simulink model "Grid_1"  (R2016b)
settings: Solver=ode3  StartTime=0.0  StopTime=10.0  RelTol=1e-3
values from neighbouring files (symbols this model uses):
  Ts = 80e-6*2    (= 0.00016)    [initSimScript.m]
undefined symbols (not defined in the file or in its folder): DiscIntNeverNeededParam
libraries: cables_lib x21, simulink x18, modbus_lib x15, powerlib x10, dynamic_load_lib x8, transformer_lib x6, discretizing x4
(part 2 of 3)

== system Grid_1/GenSet_1MVA_09082015/Simulated Generator Controller 900 kW/PQ control ==
  P_ref (pu) : Inport
  P (pu) : Inport  Port=2
  Q_ref (pu) : Inport  Port=3
  Q (pu) : Inport  Port=4
  Discrete PID Controller : simulink/Continuous/PID Controller  Controller=PID  TimeDomain=Discrete-time  SampleTime=-1  IntegratorMethod=Forward Euler  FilterMethod=Forward Euler  Form=Parallel  UseFilter=on  ControllerParametersSource=internal  P=0.001  I=1  D=0  N=10  InitialConditionSource=internal  InitialConditionForIntegrator=0  InitialConditionForFilter=0  ExternalReset=none  LimitOutput=on  UpperSaturationLimit=1.15  LowerSaturationLimit=0.85  LinearizeAsGain=off  AntiWindupMode=back-calculation  Kb=1  TrackingMode=off  Kt=1  PParamMin=[]  PParamMax=[]  IParamMin=[]  IParamMax=[]  DParamMin=[]  DParamMax=[]  NParamMin=[]  NParamMax=[]  KbParamMin=[]  KbParamMax=[]  KtParamMin=[]  KtParamMax=[]  POutMin=[]  POutMax=[]  IOutMin=[]  IOutMax=[]  DOutMin=[]  DOutMax=[]  NOutMin=[]  NOutMax=[]  KbOutMin=[]  KbOutMax=[]  KtOutMin=[]  KtOutMax=[]  IntegratorOutMin=[]  IntegratorOutMax=[]  FilterOutMin=[]  FilterOutMax=[]  SumOutMin=[]  SumOutMax=[]  SumI1OutMin=[]  SumI1OutMax=[]  SumI2OutMin=[]  SumI2OutMax=[]  SumI3OutMin=[]  SumI3OutMax=[]  SumDOutMin=[]  SumDOutMax=[]  SaturationOutMin=[]  SaturationOutMax=[]  IntegratorContinuousStateAttributes=''  IntegratorStateMustResolveToSignalObject=off  IntegratorRTWStateStorageClass=Auto  FilterContinuousStateAttributes=''  FilterStateMustResolveToSignalObject=off  FilterRTWStateStorageClass=Auto  DifferentiatorICPrevScaledInput=0  DifferentiatorOutMin=[]  DifferentiatorOutMax=[]
  Discrete PID Controller1 : simulink/Continuous/PID Controller  Controller=PID  TimeDomain=Discrete-time  SampleTime=-1  IntegratorMethod=Forward Euler  FilterMethod=Forward Euler  Form=Parallel  UseFilter=on  ControllerParametersSource=internal  P=1.2  I=2.5  D=0  N=10  InitialConditionSource=internal  InitialConditionForIntegrator=0  InitialConditionForFilter=0  ExternalReset=none  LimitOutput=on  UpperSaturationLimit=1.15  LowerSaturationLimit=0.85  LinearizeAsGain=off  AntiWindupMode=back-calculation  Kb=1  TrackingMode=off  Kt=1  PParamMin=[]  PParamMax=[]  IParamMin=[]  IParamMax=[]  DParamMin=[]  DParamMax=[]  NParamMin=[]  NParamMax=[]  KbParamMin=[]  KbParamMax=[]  KtParamMin=[]  KtParamMax=[]  POutMin=[]  POutMax=[]  IOutMin=[]  IOutMax=[]  DOutMin=[]  DOutMax=[]  NOutMin=[]  NOutMax=[]  KbOutMin=[]  KbOutMax=[]  KtOutMin=[]  KtOutMax=[]  IntegratorOutMin=[]  IntegratorOutMax=[]  FilterOutMin=[]  FilterOutMax=[]  SumOutMin=[]  SumOutMax=[]  SumI1OutMin=[]  SumI1OutMax=[]  SumI2OutMin=[]  SumI2OutMax=[]  SumI3OutMin=[]  SumI3OutMax=[]  SumDOutMin=[]  SumDOutMax=[]  SaturationOutMin=[]  SaturationOutMax=[]  IntegratorContinuousStateAttributes=''  IntegratorStateMustResolveToSignalObject=off  IntegratorRTWStateStorageClass=Auto  FilterContinuousStateAttributes=''  FilterStateMustResolveToSignalObject=off  FilterRTWStateStorageClass=Auto  DifferentiatorICPrevScaledInput=0  DifferentiatorOutMin=[]  DifferentiatorOutMax=[]
  Sum : Sum  Inputs=|-+
  Sum1 : Sum  Inputs=|-+
  w_ref (pu) : Outport
  V_ref (pu) : Outport  Port=2
  wires:
  Q_ref (pu)/1 -> Sum1/2
  Discrete PID Controller1/1 -> V_ref (pu)/1
  Q (pu)/1 -> Sum1/1
  Sum1/1 -> Discrete PID Controller1/1
  P_ref (pu)/1 -> Sum/2
  Discrete PID Controller/1 -> w_ref (pu)/1
  P (pu)/1 -> Sum/1
  Sum/1 -> Discrete PID Controller/1

== system Grid_1/GenSet_1MVA_09082015/Simulated Generator Controller 900 kW/PV control ==
  P_ref (pu) : Inport
  P (pu) : Inport  Port=2
  Discrete PID Controller : simulink/Continuous/PID Controller  Controller=PID  TimeDomain=Discrete-time  SampleTime=-1  IntegratorMethod=Forward Euler  FilterMethod=Forward Euler  Form=Parallel  UseFilter=on  ControllerParametersSource=internal  P=0.001  I=1  D=0  N=10  InitialConditionSource=internal  InitialConditionForIntegrator=0  InitialConditionForFilter=0  ExternalReset=none  LimitOutput=on  UpperSaturationLimit=1.15  LowerSaturationLimit=0.85  LinearizeAsGain=off  AntiWindupMode=back-calculation  Kb=1  TrackingMode=off  Kt=1  PParamMin=[]  PParamMax=[]  IParamMin=[]  IParamMax=[]  DParamMin=[]  DParamMax=[]  NParamMin=[]  NParamMax=[]  KbParamMin=[]  KbParamMax=[]  KtParamMin=[]  KtParamMax=[]  POutMin=[]  POutMax=[]  IOutMin=[]  IOutMax=[]  DOutMin=[]  DOutMax=[]  NOutMin=[]  NOutMax=[]  KbOutMin=[]  KbOutMax=[]  KtOutMin=[]  KtOutMax=[]  IntegratorOutMin=[]  IntegratorOutMax=[]  FilterOutMin=[]  FilterOutMax=[]  SumOutMin=[]  SumOutMax=[]  SumI1OutMin=[]  SumI1OutMax=[]  SumI2OutMin=[]  SumI2OutMax=[]  SumI3OutMin=[]  SumI3OutMax=[]  SumDOutMin=[]  SumDOutMax=[]  SaturationOutMin=[]  SaturationOutMax=[]  IntegratorContinuousStateAttributes=''  IntegratorStateMustResolveToSignalObject=off  IntegratorRTWStateStorageClass=Auto  FilterContinuousStateAttributes=''  FilterStateMustResolveToSignalObject=off  FilterRTWStateStorageClass=Auto  DifferentiatorICPrevScaledInput=0  DifferentiatorOutMin=[]  DifferentiatorOutMax=[]
  Sum : Sum  Inputs=|-+
  w_ref (pu) : Outport
  wires:
  Sum/1 -> Discrete PID Controller/1
  P (pu)/1 -> Sum/1
  Discrete PID Controller/1 -> w_ref (pu)/1
  P_ref (pu)/1 -> Sum/2

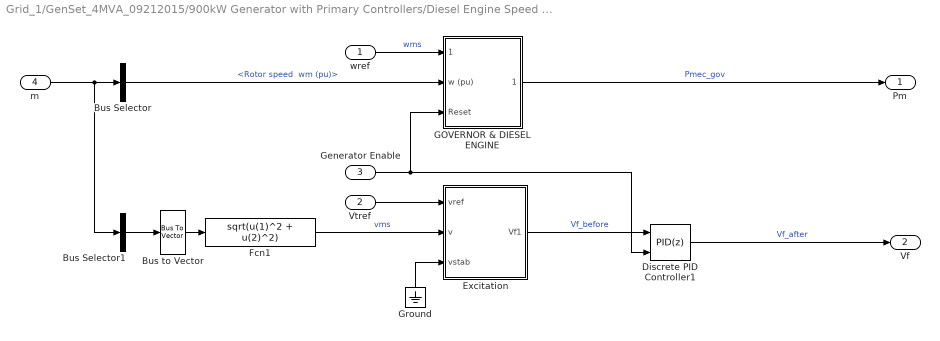
== system Grid_1/GenSet_4MVA_09212015/900kW Generator with Primary Controllers/Diesel Engine Speed & Voltage Control fast ==
  wref : Inport  SampleTime=Ts
  Vtref : Inport  Port=2  SampleTime=Ts
  Generator Enable : Inport  Port=3  SampleTime=Ts
  m : Inport  Port=4  SampleTime=Ts
  Bus Selector : BusSelector  OutputSignals="Mechanical.Rotor speed  wm (pu)"
  Bus Selector1 : BusSelector  OutputSignals="dq0 components.Stator voltage  vd (pu),dq0 components.Stator voltage  vq (pu)"  OutputAsBus=on
  Bus to Vector : BusToVector
  Discrete PID Controller1 : simulink/Continuous/PID Controller  Controller=PID  TimeDomain=Discrete-time  SampleTime=-1  IntegratorMethod=Forward Euler  FilterMethod=Forward Euler  Form=Parallel  UseFilter=on  ControllerParametersSource=internal  P=1  I=0  D=0  N=100  InitialConditionSource=internal  InitialConditionForIntegrator=0  InitialConditionForFilter=0  ExternalReset=either  LimitOutput=on  UpperSaturationLimit=5  LowerSaturationLimit=-5  LinearizeAsGain=off  AntiWindupMode=none  Kb=1  TrackingMode=off  Kt=1  PParamMin=[]  PParamMax=[]  IParamMin=[]  IParamMax=[]  DParamMin=[]  DParamMax=[]  NParamMin=[]  NParamMax=[]  KbParamMin=[]  KbParamMax=[]  KtParamMin=[]  KtParamMax=[]  POutMin=[]  POutMax=[]  IOutMin=[]  IOutMax=[]  DOutMin=[]  DOutMax=[]  NOutMin=[]  NOutMax=[]  KbOutMin=[]  KbOutMax=[]  KtOutMin=[]  KtOutMax=[]  IntegratorOutMin=[]  IntegratorOutMax=[]  FilterOutMin=[]  FilterOutMax=[]  SumOutMin=[]  SumOutMax=[]  SumI1OutMin=[]  SumI1OutMax=[]  SumI2OutMin=[]  SumI2OutMax=[]  SumI3OutMin=[]  SumI3OutMax=[]  SumDOutMin=[]  SumDOutMax=[]  SaturationOutMin=[]  SaturationOutMax=[]  IntegratorContinuousStateAttributes=''  IntegratorStateMustResolveToSignalObject=off  IntegratorRTWStateStorageClass=Auto  FilterContinuousStateAttributes=''  FilterStateMustResolveToSignalObject=off  FilterRTWStateStorageClass=Auto  DifferentiatorICPrevScaledInput=0  DifferentiatorOutMin=[]  DifferentiatorOutMax=[]
  Excitation : Subsystem  mask(Excitation System){tr=20e-4, reg=[ 200 2e-3 ], exc=[ 1 0.00000001 ], tgr=[ 1e-12 1e-12 ], damp=[0 1e-12 ], sat=[], lim=[ 0 5 0 ], v0=[ 0 0 ]}
      mask prompts: tr "Low-pass filter time constant Tr:"; reg "Regulator gain and time constant [ Ka  Ta ]:"; exc "Exciter  [ Ke  Te ]:"; tgr "Transient gain reduction [ Tb  Tc ]:"; damp "Damping filter gain and time constant  [ Kf  Tf  ]:"; sat "Field saturation parameters [ A B ]:"; lim "Regulator output limits and gain [ Efmin  Efmax  Kp ]:"; v0 "Initial values of terminal voltage  and field voltage [ Vt0 Vf0 ] :"
      mask help:
      | Implements an IEEE type 1 synchronous machine voltage regulator combined
      | to an exciter.
      |
      | The output of the block is the field voltage vfd, in pu,  to be applied to the Vf
      | Simulink input of a Synchronous Machine block.
      |
      | Connect the Vd and Vq measurements signals of the Synchronous Machine block
      | (signals 9 and 10)  to  the Vd and Vq inputs of the Excitation System block.
      mask Help: helpview(psbhelp);
  Fcn1 : Fcn  Expr=sqrt(u(1)^2 + u(2)^2)
  GOVERNOR & DIESEL ENGINE : Subsystem  mask(Diesel Engine & Governor){K=10, Ta=[0.025 0.0009 0.00574], Tlim=[0 1.1], Td=0.024, Pm0=0.0005}
      mask prompts: K "Regulator gain K:"; Ta "Actuator time constants [T4 T5 T6] (s) :"; Tlim "Torque limits [Tmin Tmax] (pu) :"; Td "Engine time delay Td (s) :"; Pm0 "Initial value of mechanical power  Pm0 (pu) :"
      mask help:
      | This block implements a diesel engine and governor system:
      | 1st and 2nd inputs: Desired and actual speed (pu)
      | Output: Diesel engine mechanical power.Motor inertia should be combined with generator.
      |
      | Actuator transfer function :
      |      Ha= (1+T4.s) / [ (s (1+T5.s)(1+T6.s) ]
      | Motor :
      |      Time delay Td
      |
      | (See reference in Tutorial Session 5)
  Ground : Ground
  Pm : Outport
  Vf : Outport  Port=2
  wires:
  GOVERNOR & DIESEL ENGINE/1(Pmec (pu)) -> Pm/1  "Pmec_gov"
  Generator Enable/1 -> GOVERNOR & DIESEL ENGINE/3(Reset), Discrete PID Controller1/2
  Bus to Vector/1 -> Fcn1/1
  Bus Selector1/1 -> Bus to Vector/1
  m/1 -> Bus Selector/1, Bus Selector1/1
  Bus Selector/1 -> GOVERNOR & DIESEL ENGINE/2(w (pu))  "<Rotor speed  wm (pu)>"
  Fcn1/1 -> Excitation/2(v)  "vms"
  Ground/1 -> Excitation/3(vstab)
  Excitation/1(Vf1) -> Discrete PID Controller1/1  "Vf_before"
  Discrete PID Controller1/1 -> Vf/1  "Vf_after"
  Vtref/1 -> Excitation/1(vref)
  wref/1 -> GOVERNOR & DIESEL ENGINE/1(wref (pu))  "wms"

== system Grid_1/GenSet_4MVA_09212015/Simulated Generator Controller 3.5 MW/PQ control ==
  P_ref (pu) : Inport
  P (pu) : Inport  Port=2
  Q_ref (pu) : Inport  Port=3
  Q (pu) : Inport  Port=4
  Discrete PID Controller : simulink/Continuous/PID Controller  Controller=PID  TimeDomain=Discrete-time  SampleTime=-1  IntegratorMethod=Forward Euler  FilterMethod=Forward Euler  Form=Parallel  UseFilter=on  ControllerParametersSource=internal  P=0.025  I=1  D=0  N=10  InitialConditionSource=internal  InitialConditionForIntegrator=0  InitialConditionForFilter=0  ExternalReset=none  LimitOutput=on  UpperSaturationLimit=1.15  LowerSaturationLimit=0.85  LinearizeAsGain=off  AntiWindupMode=back-calculation  Kb=1  TrackingMode=off  Kt=1  PParamMin=[]  PParamMax=[]  IParamMin=[]  IParamMax=[]  DParamMin=[]  DParamMax=[]  NParamMin=[]  NParamMax=[]  KbParamMin=[]  KbParamMax=[]  KtParamMin=[]  KtParamMax=[]  POutMin=[]  POutMax=[]  IOutMin=[]  IOutMax=[]  DOutMin=[]  DOutMax=[]  NOutMin=[]  NOutMax=[]  KbOutMin=[]  KbOutMax=[]  KtOutMin=[]  KtOutMax=[]  IntegratorOutMin=[]  IntegratorOutMax=[]  FilterOutMin=[]  FilterOutMax=[]  SumOutMin=[]  SumOutMax=[]  SumI1OutMin=[]  SumI1OutMax=[]  SumI2OutMin=[]  SumI2OutMax=[]  SumI3OutMin=[]  SumI3OutMax=[]  SumDOutMin=[]  SumDOutMax=[]  SaturationOutMin=[]  SaturationOutMax=[]  IntegratorContinuousStateAttributes=''  IntegratorStateMustResolveToSignalObject=off  IntegratorRTWStateStorageClass=Auto  FilterContinuousStateAttributes=''  FilterStateMustResolveToSignalObject=off  FilterRTWStateStorageClass=Auto  DifferentiatorICPrevScaledInput=0  DifferentiatorOutMin=[]  DifferentiatorOutMax=[]
  Discrete PID Controller1 : simulink/Continuous/PID Controller  Controller=PID  TimeDomain=Discrete-time  SampleTime=-1  IntegratorMethod=Forward Euler  FilterMethod=Forward Euler  Form=Parallel  UseFilter=on  ControllerParametersSource=internal  P=0.2  I=1.5  D=0  N=10  InitialConditionSource=internal  InitialConditionForIntegrator=0  InitialConditionForFilter=0  ExternalReset=none  LimitOutput=on  UpperSaturationLimit=1.15  LowerSaturationLimit=0.85  LinearizeAsGain=off  AntiWindupMode=back-calculation  Kb=1  TrackingMode=off  Kt=1  PParamMin=[]  PParamMax=[]  IParamMin=[]  IParamMax=[]  DParamMin=[]  DParamMax=[]  NParamMin=[]  NParamMax=[]  KbParamMin=[]  KbParamMax=[]  KtParamMin=[]  KtParamMax=[]  POutMin=[]  POutMax=[]  IOutMin=[]  IOutMax=[]  DOutMin=[]  DOutMax=[]  NOutMin=[]  NOutMax=[]  KbOutMin=[]  KbOutMax=[]  KtOutMin=[]  KtOutMax=[]  IntegratorOutMin=[]  IntegratorOutMax=[]  FilterOutMin=[]  FilterOutMax=[]  SumOutMin=[]  SumOutMax=[]  SumI1OutMin=[]  SumI1OutMax=[]  SumI2OutMin=[]  SumI2OutMax=[]  SumI3OutMin=[]  SumI3OutMax=[]  SumDOutMin=[]  SumDOutMax=[]  SaturationOutMin=[]  SaturationOutMax=[]  IntegratorContinuousStateAttributes=''  IntegratorStateMustResolveToSignalObject=off  IntegratorRTWStateStorageClass=Auto  FilterContinuousStateAttributes=''  FilterStateMustResolveToSignalObject=off  FilterRTWStateStorageClass=Auto  DifferentiatorICPrevScaledInput=0  DifferentiatorOutMin=[]  DifferentiatorOutMax=[]
  Sum : Sum  Inputs=|-+
  Sum1 : Sum  Inputs=|-+
  w_ref (pu) : Outport
  V_ref (pu) : Outport  Port=2
  wires:
  Q_ref (pu)/1 -> Sum1/2  "ref"
  Discrete PID Controller1/1 -> V_ref (pu)/1  "v"
  Q (pu)/1 -> Sum1/1  "pu"
  Sum1/1 -> Discrete PID Controller1/1  "dq"
  P_ref (pu)/1 -> Sum/2
  Discrete PID Controller/1 -> w_ref (pu)/1
  P (pu)/1 -> Sum/1
  Sum/1 -> Discrete PID Controller/1

== system Grid_1/GenSet_4MVA_09212015/Simulated Generator Controller 3.5 MW/PV control ==
  P_ref (pu) : Inport
  P (pu) : Inport  Port=2
  Discrete PID Controller : simulink/Continuous/PID Controller  Controller=PID  TimeDomain=Discrete-time  SampleTime=-1  IntegratorMethod=Forward Euler  FilterMethod=Forward Euler  Form=Parallel  UseFilter=on  ControllerParametersSource=internal  P=0.025  I=1  D=0  N=10  InitialConditionSource=internal  InitialConditionForIntegrator=0  InitialConditionForFilter=0  ExternalReset=none  LimitOutput=on  UpperSaturationLimit=1.15  LowerSaturationLimit=0.85  LinearizeAsGain=off  AntiWindupMode=back-calculation  Kb=1  TrackingMode=off  Kt=1  PParamMin=[]  PParamMax=[]  IParamMin=[]  IParamMax=[]  DParamMin=[]  DParamMax=[]  NParamMin=[]  NParamMax=[]  KbParamMin=[]  KbParamMax=[]  KtParamMin=[]  KtParamMax=[]  POutMin=[]  POutMax=[]  IOutMin=[]  IOutMax=[]  DOutMin=[]  DOutMax=[]  NOutMin=[]  NOutMax=[]  KbOutMin=[]  KbOutMax=[]  KtOutMin=[]  KtOutMax=[]  IntegratorOutMin=[]  IntegratorOutMax=[]  FilterOutMin=[]  FilterOutMax=[]  SumOutMin=[]  SumOutMax=[]  SumI1OutMin=[]  SumI1OutMax=[]  SumI2OutMin=[]  SumI2OutMax=[]  SumI3OutMin=[]  SumI3OutMax=[]  SumDOutMin=[]  SumDOutMax=[]  SaturationOutMin=[]  SaturationOutMax=[]  IntegratorContinuousStateAttributes=''  IntegratorStateMustResolveToSignalObject=off  IntegratorRTWStateStorageClass=Auto  FilterContinuousStateAttributes=''  FilterStateMustResolveToSignalObject=off  FilterRTWStateStorageClass=Auto  DifferentiatorICPrevScaledInput=0  DifferentiatorOutMin=[]  DifferentiatorOutMax=[]
  Sum : Sum  Inputs=|-+
  w_ref (pu) : Outport
  wires:
  Sum/1 -> Discrete PID Controller/1
  P (pu)/1 -> Sum/1
  Discrete PID Controller/1 -> w_ref (pu)/1
  P_ref (pu)/1 -> Sum/2

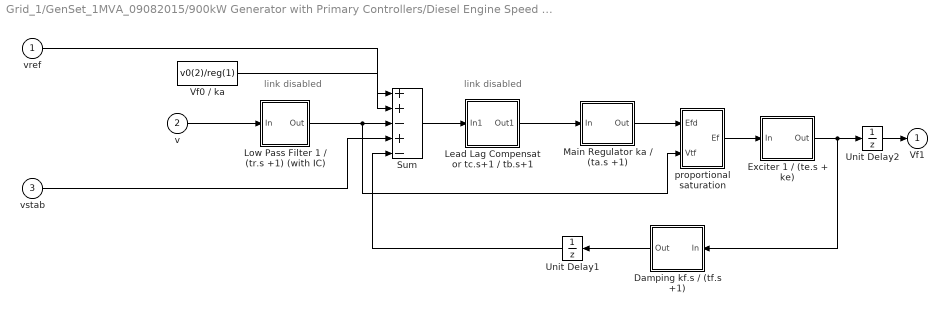
== system Grid_1/GenSet_1MVA_09082015/900kW Generator with Primary Controllers/Diesel Engine Speed & Voltage Control fast/Excitation ==
  note: link disabled
  note: link disabled
  vref : Inport
  v : Inport  Port=2
  vstab : Inport  Port=3
  Damping kf.s / (tf.s +1) : Subsystem
  Exciter 1 / (te.s + ke) : Subsystem
  Lead Lag Compensator tc.s+1 / tb.s+1 : Subsystem  AncestorBlock=|  mask(Discrete Lead-Lag Controller){T1=tgr(2), T2=tgr(1), V_Init=exc(1)*v0(2)/reg(1), Ts=Ts}
      | powerlib_extras/Discrete 
      | Control Blocks/Discrete
      | Lead-Lag
      mask prompts: T1 "Time constant T1 (s):"; T2 "Time constant T2 (s):"; V_Init "Initial input and output:"; Ts "Sample time (s):"
      mask help:
      | This block implements a discrete lead-lag controller:
      |
      |          1+T1s
      | H(s)= ------
      |          1+T2s
      |
      | States are initialized according to initial input anf output value so that simulation starts in steady state.
      mask init:
      | numc=[T1 1];
      | denc=[T2 1];
      | [Ac,Bc,Cc,Dc]=tf2ss(numc,denc);
      | 
      | %  Conversion to discrete transfer function
      | nstates = size(Ac,1);
      | invexp = inv(eye(nstates) - (Ts/2)*Ac);
      | Ad = invexp*(eye(nstates) + (Ts/2)*Ac);
      | Bd = invexp*Bc;
      | Cd = Cc*invexp*Ts;
      | Dd = Cc*invexp*Bc*(Ts/2) + Dc;
      | %
      | % Compute Initial states
      | I=eye(size(Ac));
      | x0c=inv(-Ac)*Bc*V_Init;
      | x0d=(I-Ac*Ts/2)*x0c/Ts - Bc/2*V_Init;
      | 
      | if T1==0 & T2==0, Dd=1; end
      mask Display: disp('1+T1s\n---\n1+T2s')
  Low Pass Filter 1 / (tr.s +1) (with IC) : Subsystem  AncestorBlock=|  mask(Discrete 1st-Order Filter){FilterType=Lowpass, Tc=tr, Ts=Ts, Initialize=on, Vac_Init=[0 0 60], Vdc_Init=v0(1), PlotResponse=off, param1=[1 500 0.1]}
      | powerlib_extras/Discrete 
      | Control Blocks/Discrete
      | 1st-Order
      | Discrete Filter
      mask prompts: FilterType "Filter Type:"; Tc "Time constant (s):"; Ts "Sample time:"; Initialize "Initialize filter states"; Vac_Init "AC initial input: [ Mag  Phase(degrees)  Freq(Hz) ]"; Vdc_Init "DC Initial input:"; PlotResponse "Plot filter response"; param1 "Frequency range(Hz) : [Start  End  Inc.]"
      mask init:
      | switch FilterType
      | case 1, % Lowpass
      |     X=[0 1 2 3 4];
      |     Y=[-2 -2 -3 -4 -4];
      |     numc=1;
      |     denc=[Tc 1];
      | case 2,   % Highpass
      |     X=[0 1 2 3 4];
      |     Y=[-4 -4 -3 -2 -2];
      |     numc=[1 0];
      |     denc=[1 1/Tc];
      | end
      | %
      | [Ac,Bc,Cc,Dc]=tf2ss(numc,denc);
      | %
      | %  Conversion to discrete transfer function
      | nstates = size(Ac,1);
      | invexp = inv(eye(nstates) - (Ts/2)*Ac);
      | Ad = invexp*(eye(nstates) + (Ts/2)*Ac);
      | Bd = invexp*Bc;
      | Cd = Cc*invexp*Ts;
      | Dd = Cc*invexp*Bc*(Ts/2) + Dc;
      | %
      | if Initialize==1  % Compute initial conditions on states
      |     u1=Vac_Init(1)*exp(j*Vac_Init(2)*pi/180);
      |     u2=Vdc_Init*exp(j*90*pi/180);
      |     u=u1+u2;
      |     u0=imag(u); % input at  t=0;
      |     I=eye(size(Ac));
      |     sI1=I*j*(2*pi*Vac_Init(3));
      |     sI2=I*j*0;
      |     x=inv(sI1-Ac)*Bc*u1 + inv(sI2-Ac)*Bc*u2;
      |     x0c=imag(x);
      |     x0d=(I-Ac*Ts/2)*x0c/Ts - Bc/2*u0;
      | else
      |     x0d=0;
      | end
      | 
      | %
      | if PlotResponse==1 % Plot frequency and step response
      |     figure(1)
      |     sys=ss(Ad,Bd,Cd,Dd,Ts);
      |     f=param1(1):param1(3):param1(2);
      |     w=2*pi*f;
      |     [mag phase]=bode(sys,w);
      |     subplot(2,1,1)
      |     plot(f,squeeze(mag))
      |     title('Magnitude')
      |     grid
      |     subplot(2,1,2)
      |     plot(f,squeeze(phase))
      |     title('Phase (degrees)')
      |     xlabel('Hz')
      |     grid
      |     figure(2)
      |     step(sys)
      | end
      mask TypeOptions FilterType: Lowpass | Highpass
      mask Callback Initialize: p4=get_param(gcb,'Initialize');if strcmp(p4,'on');visible={'on','on','on','on','on','on','on',get_param(gcb,'PlotResponse')};else;visible={'on','on','on','on','off','off','on',get_param(gcb,'PlotResponse')};end;set_param(gcb,'MaskVisibilities',visible)
      mask Callback PlotResponse: p7=get_param(gcb,'PlotResponse');if strcmp(p7,'on');visible={'on','on','on','on',get_param(gcb,'Initialize'),get_param(gcb,'Initialize'),'on','on'};else;visible={'on','on','on','on',get_param(gcb,'Initialize'),get_param(gcb,'Initialize'),'on','off'};end;set_param(gcb,'MaskVisibilities',visible)
      mask Display: plot(X,Y);
  Main Regulator ka / (ta.s +1) : Subsystem
  Sum : Sum  Inputs=++-+-  SaturateOnIntegerOverflow=on  InputSameDT=on  OutDataTypeStr=Inherit: Same as first input
  Unit Delay1 : UnitDelay  SampleTime=Ts
  Unit Delay2 : UnitDelay  InitialCondition=v0(2)  SampleTime=Ts
  Vf0 / ka : Constant  Value=v0(2)/reg(1)
  proportional saturation : Subsystem
  Vf1 : Outport
  wires:
  Exciter 1 / (te.s + ke)/1(Out) -> Damping kf.s / (tf.s +1)/1(In), Unit Delay2/1
  Damping kf.s / (tf.s +1)/1(Out) -> Unit Delay1/1
  Main Regulator ka / (ta.s +1)/1(Out) -> proportional saturation/1(Efd)
  Vf0 / ka/1 -> Sum/2
  Low Pass Filter 1 / (tr.s +1) (with IC)/1(Out) -> Sum/3, proportional saturation/2(Vtf)
  vstab/1 -> Sum/4
  vref/1 -> Sum/1
  v/1 -> Low Pass Filter 1 / (tr.s +1) (with IC)/1(In)
  Sum/1 -> Lead Lag Compensator tc.s+1 / tb.s+1/1(In1)
  Lead Lag Compensator tc.s+1 / tb.s+1/1(Out1) -> Main Regulator ka / (ta.s +1)/1(In)
  proportional saturation/1(Ef) -> Exciter 1 / (te.s + ke)/1(In)
  Unit Delay1/1 -> Sum/5
  Unit Delay2/1 -> Vf1/1

== system Grid_1/GenSet_1MVA_09082015/900kW Generator with Primary Controllers/Diesel Engine Speed & Voltage Control fast/GOVERNOR & DIESEL ENGINE ==
  note: ACTUATOR
  wref (pu) : Inport
  w (pu) : Inport  Port=2
  Reset : Inport  Port=3
  Discrete PID Controller : simulink/Continuous/PID Controller  Controller=PD  TimeDomain=Discrete-time  SampleTime=-1  IntegratorMethod=Forward Euler  FilterMethod=Forward Euler  Form=Parallel  UseFilter=on  ControllerParametersSource=internal  P=1  I=0  D=0.5  N=10000  InitialConditionSource=internal  InitialConditionForIntegrator=0  InitialConditionForFilter=0  ExternalReset=rising  ZeroCross=off  LimitOutput=off  UpperSaturationLimit=.5  LowerSaturationLimit=-.5  LinearizeAsGain=off  AntiWindupMode=none  Kb=1  TrackingMode=off  Kt=1  PParamMin=[]  PParamMax=[]  IParamMin=[]  IParamMax=[]  DParamMin=[]  DParamMax=[]  NParamMin=[]  NParamMax=[]  KbParamMin=[]  KbParamMax=[]  KtParamMin=[]  KtParamMax=[]  POutMin=[]  POutMax=[]  IOutMin=[]  IOutMax=[]  DOutMin=[]  DOutMax=[]  NOutMin=[]  NOutMax=[]  KbOutMin=[]  KbOutMax=[]  KtOutMin=[]  KtOutMax=[]  IntegratorOutMin=[]  IntegratorOutMax=[]  FilterOutMin=[]  FilterOutMax=[]  SumOutMin=[]  SumOutMax=[]  SumI1OutMin=[]  SumI1OutMax=[]  SumI2OutMin=[]  SumI2OutMax=[]  SumI3OutMin=[]  SumI3OutMax=[]  SumDOutMin=[]  SumDOutMax=[]  SaturationOutMin=[]  SaturationOutMax=[]  IntegratorContinuousStateAttributes=''  IntegratorStateMustResolveToSignalObject=off  IntegratorRTWStateStorageClass=Auto  FilterContinuousStateAttributes=''  FilterStateMustResolveToSignalObject=off  FilterRTWStateStorageClass=Auto  DifferentiatorICPrevScaledInput=0  DifferentiatorOutMin=[]  DifferentiatorOutMax=[]
  Discrete-Time Integrator : DiscreteIntegrator  IntegratorMethod=Integration: Backward Euler  ExternalReset=either  InitialCondition=Pm0  SampleTime=-1  LimitOutput=on  UpperSaturationLimit=Tlim(2)  LowerSaturationLimit=Tlim(1)  ICPrevOutput=DiscIntNeverNeededParam  ICPrevScaledInput=DiscIntNeverNeededParam
  ENGINE Td1 : TransportDelay  Commented=on  DelayTime=Td  InitialOutput=Pm0  BufferSize=7168
  Engine Delay : Delay  DelayLength=ceil(Td/Ts)  InitialCondition=Pm0
  Gain K : Gain  Gain=K  SaturateOnIntegerOverflow=on  OutDataTypeStr=Inherit: Same as input  ParamDataTypeStr=Inherit: Same as input
  Product : Product  SaturateOnIntegerOverflow=on  InputSameDT=on  OutDataTypeStr=Inherit: Same as first input
  Sum : Sum  Inputs=+-  SaturateOnIntegerOverflow=on  InputSameDT=on  OutDataTypeStr=Inherit: Same as first input
  TF3 : discretizing/Discretized Transfer Fcn  Numerator=1  Denominator=([Ta(3) 1])  AbsTol=auto  SampleTime=Ts  method=zoh  Wc=1
  TF4 : discretizing/Discretized Transfer Fcn  Numerator=([Ta(1) 1])  Denominator=([Ta(2) 1])  AbsTol=auto  SampleTime=Ts  method=zoh  Wc=1
  Pmec (pu) : Outport
  wires:
  Discrete PID Controller/1 -> Gain K/1
  Sum/1 -> Discrete PID Controller/1
  Gain K/1 -> TF4/1
  w (pu)/1 -> Product/2, Sum/2
  Engine Delay/1 -> Product/1
  wref (pu)/1 -> Sum/1
  Product/1 -> Pmec (pu)/1
  Discrete-Time Integrator/1 -> Engine Delay/1  "Torque"
  TF3/1 -> Discrete-Time Integrator/1
  TF4/1 -> TF3/1
  Reset/1 -> Discrete-Time Integrator/2, Discrete PID Controller/2

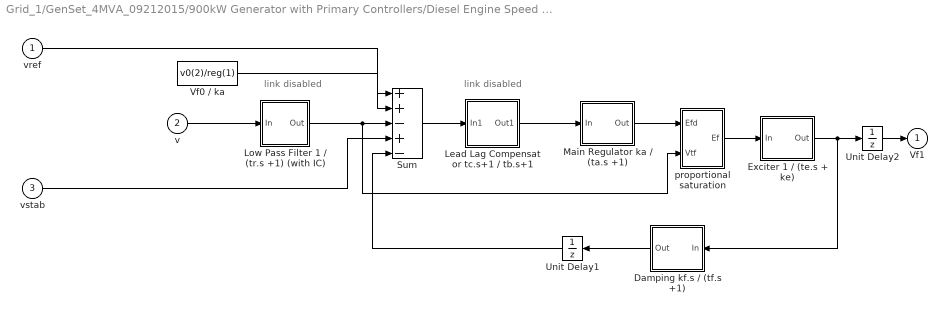
== system Grid_1/GenSet_4MVA_09212015/900kW Generator with Primary Controllers/Diesel Engine Speed & Voltage Control fast/Excitation ==
  note: link disabled
  note: link disabled
  vref : Inport
  v : Inport  Port=2
  vstab : Inport  Port=3
  Damping kf.s / (tf.s +1) : Subsystem
  Exciter 1 / (te.s + ke) : Subsystem
  Lead Lag Compensator tc.s+1 / tb.s+1 : Subsystem  AncestorBlock=|  mask(Discrete Lead-Lag Controller){T1=tgr(2), T2=tgr(1), V_Init=exc(1)*v0(2)/reg(1), Ts=Ts}
      | powerlib_extras/Discrete 
      | Control Blocks/Discrete
      | Lead-Lag
      mask prompts: T1 "Time constant T1 (s):"; T2 "Time constant T2 (s):"; V_Init "Initial input and output:"; Ts "Sample time (s):"
      mask help:
      | This block implements a discrete lead-lag controller:
      |
      |          1+T1s
      | H(s)= ------
      |          1+T2s
      |
      | States are initialized according to initial input anf output value so that simulation starts in steady state.
      mask init: same as Grid_1/GenSet_1MVA_09082015/900kW Generator with Primary Controllers/Diesel Engine Speed & Voltage Control fast/Excitation/Lead Lag Compensator tc.s+1 / tb.s+1
      mask Display: disp('1+T1s\n---\n1+T2s')
  Low Pass Filter 1 / (tr.s +1) (with IC) : Subsystem  AncestorBlock=|  mask(Discrete 1st-Order Filter){FilterType=Lowpass, Tc=tr, Ts=Ts, Initialize=on, Vac_Init=[0 0 60], Vdc_Init=v0(1), PlotResponse=off, param1=[1 500 0.1]}
      | powerlib_extras/Discrete 
      | Control Blocks/Discrete
      | 1st-Order
      | Discrete Filter
      mask prompts: FilterType "Filter Type:"; Tc "Time constant (s):"; Ts "Sample time:"; Initialize "Initialize filter states"; Vac_Init "AC initial input: [ Mag  Phase(degrees)  Freq(Hz) ]"; Vdc_Init "DC Initial input:"; PlotResponse "Plot filter response"; param1 "Frequency range(Hz) : [Start  End  Inc.]"
      mask init: same as Grid_1/GenSet_1MVA_09082015/900kW Generator with Primary Controllers/Diesel Engine Speed & Voltage Control fast/Excitation/Low Pass Filter 1 / (tr.s +1) (with IC)
      mask TypeOptions FilterType: Lowpass | Highpass
      mask Callback Initialize: p4=get_param(gcb,'Initialize');if strcmp(p4,'on');visible={'on','on','on','on','on','on','on',get_param(gcb,'PlotResponse')};else;visible={'on','on','on','on','off','off','on',get_param(gcb,'PlotResponse')};end;set_param(gcb,'MaskVisibilities',visible)
      mask Callback PlotResponse: p7=get_param(gcb,'PlotResponse');if strcmp(p7,'on');visible={'on','on','on','on',get_param(gcb,'Initialize'),get_param(gcb,'Initialize'),'on','on'};else;visible={'on','on','on','on',get_param(gcb,'Initialize'),get_param(gcb,'Initialize'),'on','off'};end;set_param(gcb,'MaskVisibilities',visible)
      mask Display: plot(X,Y);
  Main Regulator ka / (ta.s +1) : Subsystem
  Sum : Sum  Inputs=++-+-  SaturateOnIntegerOverflow=on  InputSameDT=on  OutDataTypeStr=Inherit: Same as first input
  Unit Delay1 : UnitDelay  SampleTime=Ts
  Unit Delay2 : UnitDelay  InitialCondition=v0(2)  SampleTime=Ts
  Vf0 / ka : Constant  Value=v0(2)/reg(1)
  proportional saturation : Subsystem
  Vf1 : Outport
  wires:
  Unit Delay2/1 -> Vf1/1
  Unit Delay1/1 -> Sum/5
  proportional saturation/1(Ef) -> Exciter 1 / (te.s + ke)/1(In)
  Lead Lag Compensator tc.s+1 / tb.s+1/1(Out1) -> Main Regulator ka / (ta.s +1)/1(In)
  Sum/1 -> Lead Lag Compensator tc.s+1 / tb.s+1/1(In1)
  v/1 -> Low Pass Filter 1 / (tr.s +1) (with IC)/1(In)
  vref/1 -> Sum/1
  vstab/1 -> Sum/4
  Low Pass Filter 1 / (tr.s +1) (with IC)/1(Out) -> proportional saturation/2(Vtf), Sum/3
  Vf0 / ka/1 -> Sum/2
  Main Regulator ka / (ta.s +1)/1(Out) -> proportional saturation/1(Efd)
  Damping kf.s / (tf.s +1)/1(Out) -> Unit Delay1/1
  Exciter 1 / (te.s + ke)/1(Out) -> Unit Delay2/1, Damping kf.s / (tf.s +1)/1(In)

== system Grid_1/GenSet_4MVA_09212015/900kW Generator with Primary Controllers/Diesel Engine Speed & Voltage Control fast/GOVERNOR & DIESEL ENGINE ==
  note: ACTUATOR
  wref (pu) : Inport
  w (pu) : Inport  Port=2
  Reset : Inport  Port=3
  Discrete PID Controller : simulink/Continuous/PID Controller  Controller=PD  TimeDomain=Discrete-time  SampleTime=-1  IntegratorMethod=Forward Euler  FilterMethod=Forward Euler  Form=Parallel  UseFilter=on  ControllerParametersSource=internal  P=1  I=0  D=0.5  N=10000  InitialConditionSource=internal  InitialConditionForIntegrator=0  InitialConditionForFilter=0  ExternalReset=rising  ZeroCross=off  LimitOutput=off  UpperSaturationLimit=.5  LowerSaturationLimit=-.5  LinearizeAsGain=off  AntiWindupMode=none  Kb=1  TrackingMode=off  Kt=1  PParamMin=[]  PParamMax=[]  IParamMin=[]  IParamMax=[]  DParamMin=[]  DParamMax=[]  NParamMin=[]  NParamMax=[]  KbParamMin=[]  KbParamMax=[]  KtParamMin=[]  KtParamMax=[]  POutMin=[]  POutMax=[]  IOutMin=[]  IOutMax=[]  DOutMin=[]  DOutMax=[]  NOutMin=[]  NOutMax=[]  KbOutMin=[]  KbOutMax=[]  KtOutMin=[]  KtOutMax=[]  IntegratorOutMin=[]  IntegratorOutMax=[]  FilterOutMin=[]  FilterOutMax=[]  SumOutMin=[]  SumOutMax=[]  SumI1OutMin=[]  SumI1OutMax=[]  SumI2OutMin=[]  SumI2OutMax=[]  SumI3OutMin=[]  SumI3OutMax=[]  SumDOutMin=[]  SumDOutMax=[]  SaturationOutMin=[]  SaturationOutMax=[]  IntegratorContinuousStateAttributes=''  IntegratorStateMustResolveToSignalObject=off  IntegratorRTWStateStorageClass=Auto  FilterContinuousStateAttributes=''  FilterStateMustResolveToSignalObject=off  FilterRTWStateStorageClass=Auto  DifferentiatorICPrevScaledInput=0  DifferentiatorOutMin=[]  DifferentiatorOutMax=[]
  Discrete-Time Integrator : DiscreteIntegrator  IntegratorMethod=Integration: Backward Euler  ExternalReset=either  InitialCondition=Pm0  SampleTime=-1  LimitOutput=on  UpperSaturationLimit=Tlim(2)  LowerSaturationLimit=Tlim(1)  ICPrevOutput=DiscIntNeverNeededParam  ICPrevScaledInput=DiscIntNeverNeededParam
  Engine Delay : Delay  DelayLength=ceil(Td/Ts)  InitialCondition=Pm0
  Gain K : Gain  Gain=K  SaturateOnIntegerOverflow=on  OutDataTypeStr=Inherit: Same as input  ParamDataTypeStr=Inherit: Same as input
  Product : Product  SaturateOnIntegerOverflow=on  InputSameDT=on  OutDataTypeStr=Inherit: Same as first input
  Sum : Sum  Inputs=+-  SaturateOnIntegerOverflow=on  InputSameDT=on  OutDataTypeStr=Inherit: Same as first input
  TF3 : discretizing/Discretized Transfer Fcn  Numerator=1  Denominator=([Ta(3) 1])  AbsTol=auto  SampleTime=Ts  method=zoh  Wc=1
  TF4 : discretizing/Discretized Transfer Fcn  Numerator=([Ta(1) 1])  Denominator=([Ta(2) 1])  AbsTol=auto  SampleTime=Ts  method=zoh  Wc=1
  Pmec (pu) : Outport
  wires:
  Reset/1 -> Discrete PID Controller/2, Discrete-Time Integrator/2
  TF4/1 -> TF3/1
  TF3/1 -> Discrete-Time Integrator/1
  Discrete-Time Integrator/1 -> Engine Delay/1  "Torque"
  Product/1 -> Pmec (pu)/1
  wref (pu)/1 -> Sum/1
  Engine Delay/1 -> Product/1
  w (pu)/1 -> Sum/2, Product/2
  Gain K/1 -> TF4/1
  Sum/1 -> Discrete PID Controller/1
  Discrete PID Controller/1 -> Gain K/1

== system Grid_1/GenSet_1MVA_09082015/900kW Generator with Primary Controllers/Diesel Engine Speed & Voltage Control fast/Excitation/Damping kf.s // (tf.s +1) ==
  note: link disabled
  In : Inport
  1st-Order Discrete Filter : Subsystem  AncestorBlock=|  mask(Discrete 1st-Order Filter){FilterType=Highpass, Tc=damp(2), Ts=Ts, Initialize=on, Vac_Init=[0 0 60], Vdc_Init=damp(1)*v0(2)/damp(2), PlotResponse=off, param1=[1 500 0.1]}
      | powerlib_extras/Discrete 
      | Control Blocks/Discrete
      | 1st-Order
      | Discrete Filter
      mask prompts: FilterType "Filter Type:"; Tc "Time constant (s):"; Ts "Sample time:"; Initialize "Initialize filter states"; Vac_Init "AC initial input: [ Mag  Phase(degrees)  Freq(Hz) ]"; Vdc_Init "DC Initial input:"; PlotResponse "Plot filter response"; param1 "Frequency range(Hz) : [Start  End  Inc.]"
      mask init: same as Grid_1/GenSet_1MVA_09082015/900kW Generator with Primary Controllers/Diesel Engine Speed & Voltage Control fast/Excitation/Low Pass Filter 1 / (tr.s +1) (with IC)
      mask TypeOptions FilterType: Lowpass | Highpass
      mask Callback Initialize: p4=get_param(gcb,'Initialize');if strcmp(p4,'on');visible={'on','on','on','on','on','on','on',get_param(gcb,'PlotResponse')};else;visible={'on','on','on','on','off','off','on',get_param(gcb,'PlotResponse')};end;set_param(gcb,'MaskVisibilities',visible)
      mask Callback PlotResponse: p7=get_param(gcb,'PlotResponse');if strcmp(p7,'on');visible={'on','on','on','on',get_param(gcb,'Initialize'),get_param(gcb,'Initialize'),'on','on'};else;visible={'on','on','on','on',get_param(gcb,'Initialize'),get_param(gcb,'Initialize'),'on','off'};end;set_param(gcb,'MaskVisibilities',visible)
      mask Display: plot(X,Y);
  Gain : Gain  Gain=damp(1)/damp(2)  SaturateOnIntegerOverflow=on  OutDataTypeStr=Inherit: Same as input  ParamDataTypeStr=Inherit: Same as input
  Out : Outport
  wires:
  In/1 -> Gain/1
  Gain/1 -> 1st-Order Discrete Filter/1(In)
  1st-Order Discrete Filter/1(Out) -> Out/1

== system Grid_1/GenSet_1MVA_09082015/900kW Generator with Primary Controllers/Diesel Engine Speed & Voltage Control fast/Excitation/Exciter 1 // (te.s + ke) ==
  note: link disabled
  In : Inport
  1st order Lowpass : Subsystem  AncestorBlock=|  mask(Discrete 1st-Order Filter){FilterType=Lowpass, Tc=exc(2)/exc(1), Ts=Ts, Initialize=on, Vac_Init=[0.0 0 60], Vdc_Init=v0(2), PlotResponse=off, param1=[1 500 0.1]}
      | powerlib_extras/Discrete 
      | Control Blocks/Discrete
      | 1st-Order
      | Discrete Filter
      mask prompts: FilterType "Filter Type:"; Tc "Time constant (s):"; Ts "Sample time:"; Initialize "Initialize filter states"; Vac_Init "AC initial input: [ Mag  Phase(degrees)  Freq(Hz) ]"; Vdc_Init "DC Initial input:"; PlotResponse "Plot filter response"; param1 "Frequency range(Hz) : [Start  End  Inc.]"
      mask init: same as Grid_1/GenSet_1MVA_09082015/900kW Generator with Primary Controllers/Diesel Engine Speed & Voltage Control fast/Excitation/Low Pass Filter 1 / (tr.s +1) (with IC)
      mask TypeOptions FilterType: Lowpass | Highpass
      mask Callback Initialize: p4=get_param(gcb,'Initialize');if strcmp(p4,'on');visible={'on','on','on','on','on','on','on',get_param(gcb,'PlotResponse')};else;visible={'on','on','on','on','off','off','on',get_param(gcb,'PlotResponse')};end;set_param(gcb,'MaskVisibilities',visible)
      mask Callback PlotResponse: p7=get_param(gcb,'PlotResponse');if strcmp(p7,'on');visible={'on','on','on','on',get_param(gcb,'Initialize'),get_param(gcb,'Initialize'),'on','on'};else;visible={'on','on','on','on',get_param(gcb,'Initialize'),get_param(gcb,'Initialize'),'on','off'};end;set_param(gcb,'MaskVisibilities',visible)
      mask Display: plot(X,Y);
  Gain : Gain  Gain=1/exc(1)  SaturateOnIntegerOverflow=on  OutDataTypeStr=Inherit: Same as input  ParamDataTypeStr=Inherit: Same as input
  Out : Outport
  wires:
  1st order Lowpass/1(Out) -> Out/1
  In/1 -> Gain/1
  Gain/1 -> 1st order Lowpass/1(In)

== system Grid_1/GenSet_1MVA_09082015/900kW Generator with Primary Controllers/Diesel Engine Speed & Voltage Control fast/Excitation/Lead Lag Compensator tc.s+1 // tb.s+1 ==
  In1 : Inport
  Discrete State-Space : DiscreteStateSpace  A=Ad  B=Bd  C=Cd  D=Dd  X0=x0d  SampleTime=Ts
  Out1 : Outport
  wires:
  Discrete State-Space/1 -> Out1/1
  In1/1 -> Discrete State-Space/1

== system Grid_1/GenSet_1MVA_09082015/900kW Generator with Primary Controllers/Diesel Engine Speed & Voltage Control fast/Excitation/Low Pass Filter 1 // (tr.s +1) (with IC) ==
  In : Inport
  Discrete State-Space : DiscreteStateSpace  A=Ad  B=Bd  C=Cd  D=Dd  X0=x0d  SampleTime=Ts
  Out : Outport
  wires:
  Discrete State-Space/1 -> Out/1
  In/1 -> Discrete State-Space/1

== system Grid_1/GenSet_1MVA_09082015/900kW Generator with Primary Controllers/Diesel Engine Speed & Voltage Control fast/Excitation/Main Regulator ka // (ta.s +1) ==
  note: link disabled
  In : Inport
  1st order Lowpass : Subsystem  AncestorBlock=|  mask(Discrete 1st-Order Filter){FilterType=Lowpass, Tc=reg(2), Ts=Ts, Initialize=on, Vac_Init=[0.0 0 60], Vdc_Init=exc(1)*v0(2), PlotResponse=off, param1=[1 500 0.1]}
      | powerlib_extras/Discrete 
      | Control Blocks/Discrete
      | 1st-Order
      | Discrete Filter
      mask prompts: FilterType "Filter Type:"; Tc "Time constant (s):"; Ts "Sample time:"; Initialize "Initialize filter states"; Vac_Init "AC initial input: [ Mag  Phase(degrees)  Freq(Hz) ]"; Vdc_Init "DC Initial input:"; PlotResponse "Plot filter response"; param1 "Frequency range(Hz) : [Start  End  Inc.]"
      mask init: same as Grid_1/GenSet_1MVA_09082015/900kW Generator with Primary Controllers/Diesel Engine Speed & Voltage Control fast/Excitation/Low Pass Filter 1 / (tr.s +1) (with IC)
      mask TypeOptions FilterType: Lowpass | Highpass
      mask Callback Initialize: p4=get_param(gcb,'Initialize');if strcmp(p4,'on');visible={'on','on','on','on','on','on','on',get_param(gcb,'PlotResponse')};else;visible={'on','on','on','on','off','off','on',get_param(gcb,'PlotResponse')};end;set_param(gcb,'MaskVisibilities',visible)
      mask Callback PlotResponse: p7=get_param(gcb,'PlotResponse');if strcmp(p7,'on');visible={'on','on','on','on',get_param(gcb,'Initialize'),get_param(gcb,'Initialize'),'on','on'};else;visible={'on','on','on','on',get_param(gcb,'Initialize'),get_param(gcb,'Initialize'),'on','off'};end;set_param(gcb,'MaskVisibilities',visible)
      mask Display: plot(X,Y);
  Gain : Gain  Gain=reg(1)  SaturateOnIntegerOverflow=on  OutDataTypeStr=Inherit: Same as input  ParamDataTypeStr=Inherit: Same as input
  Out : Outport
  wires:
  Gain/1 -> 1st order Lowpass/1(In)
  In/1 -> Gain/1
  1st order Lowpass/1(Out) -> Out/1

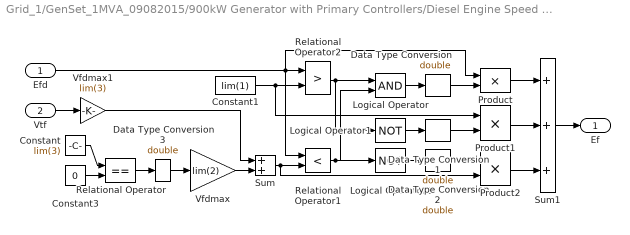
== system Grid_1/GenSet_1MVA_09082015/900kW Generator with Primary Controllers/Diesel Engine Speed & Voltage Control fast/Excitation/proportional saturation ==
  Efd : Inport
  Vtf : Inport  Port=2
  Constant : Constant  Value=lim(3)
  Constant1 : Constant  Value=lim(1)
  Constant3 : Constant  Value=0
  Data Type Conversion{,1..3} (4 alike) : DataTypeConversion  OutDataTypeStr=double  SaturateOnIntegerOverflow=on  RndMeth=Zero
  Logical Operator : Logic
  Logical Operator1 : Logic  Operator=NOT  Inputs=1
  Logical Operator2 : Logic  Operator=NOT  Inputs=1
  Product : Product  SaturateOnIntegerOverflow=on  InputSameDT=on  OutDataTypeStr=Inherit: Same as first input
  Product1 : Product  SaturateOnIntegerOverflow=on  InputSameDT=on  OutDataTypeStr=Inherit: Same as first input
  Product2 : Product  SaturateOnIntegerOverflow=on  InputSameDT=on  OutDataTypeStr=Inherit: Same as first input
  Relational Operator : RelationalOperator  Operator===  RndMeth=Nearest  InputSameDT=on
  Relational Operator1 : RelationalOperator  Operator=<  RndMeth=Nearest  InputSameDT=on
  Relational Operator2 : RelationalOperator  Operator=>  RndMeth=Nearest  InputSameDT=on
  Sum : Sum  SaturateOnIntegerOverflow=on  InputSameDT=on  OutDataTypeStr=Inherit: Same as first input
  Sum1 : Sum  Inputs=+++  SaturateOnIntegerOverflow=on  InputSameDT=on  OutDataTypeStr=Inherit: Same as first input
  Vfdmax : Gain  Gain=lim(2)  SaturateOnIntegerOverflow=on  OutDataTypeStr=Inherit: Same as input  ParamDataTypeStr=Inherit: Same as input
  Vfdmax1 : Gain  Gain=lim(3)  SaturateOnIntegerOverflow=on  OutDataTypeStr=Inherit: Same as input  ParamDataTypeStr=Inherit: Same as input
  Ef : Outport
  wires:
  Vtf/1 -> Vfdmax1/1
  Constant/1 -> Relational Operator/1
  Constant3/1 -> Relational Operator/2
  Vfdmax/1 -> Sum/2
  Vfdmax1/1 -> Sum/1
  Sum/1 -> Product2/2, Relational Operator1/2
  Relational Operator2/1 -> Logical Operator1/1, Logical Operator/1
  Relational Operator1/1 -> Logical Operator2/1, Logical Operator/2
  Constant1/1 -> Relational Operator2/2, Product1/1
  Efd/1 -> Relational Operator2/1, Relational Operator1/1, Product/1
  Sum1/1 -> Ef/1
  Product/1 -> Sum1/1
  Product2/1 -> Sum1/3
  Product1/1 -> Sum1/2
  Logical Operator/1 -> Data Type Conversion/1
  Data Type Conversion/1 -> Product/2
  Logical Operator1/1 -> Data Type Conversion1/1
  Data Type Conversion1/1 -> Product1/2
  Logical Operator2/1 -> Data Type Conversion2/1
  Data Type Conversion2/1 -> Product2/1
  Relational Operator/1 -> Data Type Conversion3/1
  Data Type Conversion3/1 -> Vfdmax/1

== system Grid_1/GenSet_4MVA_09212015/900kW Generator with Primary Controllers/Diesel Engine Speed & Voltage Control fast/Excitation/Damping kf.s // (tf.s +1) ==
  note: link disabled
  In : Inport
  1st-Order Discrete Filter : Subsystem  AncestorBlock=|  mask(Discrete 1st-Order Filter){FilterType=Highpass, Tc=damp(2), Ts=Ts, Initialize=on, Vac_Init=[0 0 60], Vdc_Init=damp(1)*v0(2)/damp(2), PlotResponse=off, param1=[1 500 0.1]}
      | powerlib_extras/Discrete 
      | Control Blocks/Discrete
      | 1st-Order
      | Discrete Filter
      mask prompts: FilterType "Filter Type:"; Tc "Time constant (s):"; Ts "Sample time:"; Initialize "Initialize filter states"; Vac_Init "AC initial input: [ Mag  Phase(degrees)  Freq(Hz) ]"; Vdc_Init "DC Initial input:"; PlotResponse "Plot filter response"; param1 "Frequency range(Hz) : [Start  End  Inc.]"
      mask init: same as Grid_1/GenSet_1MVA_09082015/900kW Generator with Primary Controllers/Diesel Engine Speed & Voltage Control fast/Excitation/Low Pass Filter 1 / (tr.s +1) (with IC)
      mask TypeOptions FilterType: Lowpass | Highpass
      mask Callback Initialize: p4=get_param(gcb,'Initialize');if strcmp(p4,'on');visible={'on','on','on','on','on','on','on',get_param(gcb,'PlotResponse')};else;visible={'on','on','on','on','off','off','on',get_param(gcb,'PlotResponse')};end;set_param(gcb,'MaskVisibilities',visible)
      mask Callback PlotResponse: p7=get_param(gcb,'PlotResponse');if strcmp(p7,'on');visible={'on','on','on','on',get_param(gcb,'Initialize'),get_param(gcb,'Initialize'),'on','on'};else;visible={'on','on','on','on',get_param(gcb,'Initialize'),get_param(gcb,'Initialize'),'on','off'};end;set_param(gcb,'MaskVisibilities',visible)
      mask Display: plot(X,Y);
  Gain : Gain  Gain=damp(1)/damp(2)  SaturateOnIntegerOverflow=on  OutDataTypeStr=Inherit: Same as input  ParamDataTypeStr=Inherit: Same as input
  Out : Outport
  wires:
  1st-Order Discrete Filter/1(Out) -> Out/1
  Gain/1 -> 1st-Order Discrete Filter/1(In)
  In/1 -> Gain/1

== system Grid_1/GenSet_4MVA_09212015/900kW Generator with Primary Controllers/Diesel Engine Speed & Voltage Control fast/Excitation/Exciter 1 // (te.s + ke) ==
  note: link disabled
  In : Inport
  1st order Lowpass : Subsystem  AncestorBlock=|  mask(Discrete 1st-Order Filter){FilterType=Lowpass, Tc=exc(2)/exc(1), Ts=Ts, Initialize=on, Vac_Init=[0.0 0 60], Vdc_Init=v0(2), PlotResponse=off, param1=[1 500 0.1]}
      | powerlib_extras/Discrete 
      | Control Blocks/Discrete
      | 1st-Order
      | Discrete Filter
      mask prompts: FilterType "Filter Type:"; Tc "Time constant (s):"; Ts "Sample time:"; Initialize "Initialize filter states"; Vac_Init "AC initial input: [ Mag  Phase(degrees)  Freq(Hz) ]"; Vdc_Init "DC Initial input:"; PlotResponse "Plot filter response"; param1 "Frequency range(Hz) : [Start  End  Inc.]"
      mask init: same as Grid_1/GenSet_1MVA_09082015/900kW Generator with Primary Controllers/Diesel Engine Speed & Voltage Control fast/Excitation/Low Pass Filter 1 / (tr.s +1) (with IC)
      mask TypeOptions FilterType: Lowpass | Highpass
      mask Callback Initialize: p4=get_param(gcb,'Initialize');if strcmp(p4,'on');visible={'on','on','on','on','on','on','on',get_param(gcb,'PlotResponse')};else;visible={'on','on','on','on','off','off','on',get_param(gcb,'PlotResponse')};end;set_param(gcb,'MaskVisibilities',visible)
      mask Callback PlotResponse: p7=get_param(gcb,'PlotResponse');if strcmp(p7,'on');visible={'on','on','on','on',get_param(gcb,'Initialize'),get_param(gcb,'Initialize'),'on','on'};else;visible={'on','on','on','on',get_param(gcb,'Initialize'),get_param(gcb,'Initialize'),'on','off'};end;set_param(gcb,'MaskVisibilities',visible)
      mask Display: plot(X,Y);
  Gain : Gain  Gain=1/exc(1)  SaturateOnIntegerOverflow=on  OutDataTypeStr=Inherit: Same as input  ParamDataTypeStr=Inherit: Same as input
  Out : Outport
  wires:
  Gain/1 -> 1st order Lowpass/1(In)
  In/1 -> Gain/1
  1st order Lowpass/1(Out) -> Out/1

== system Grid_1/GenSet_4MVA_09212015/900kW Generator with Primary Controllers/Diesel Engine Speed & Voltage Control fast/Excitation/Lead Lag Compensator tc.s+1 // tb.s+1 ==
  In1 : Inport
  Discrete State-Space : DiscreteStateSpace  A=Ad  B=Bd  C=Cd  D=Dd  X0=x0d  SampleTime=Ts
  Out1 : Outport
  wires:
  In1/1 -> Discrete State-Space/1
  Discrete State-Space/1 -> Out1/1

== system Grid_1/GenSet_4MVA_09212015/900kW Generator with Primary Controllers/Diesel Engine Speed & Voltage Control fast/Excitation/Low Pass Filter 1 // (tr.s +1) (with IC) ==
  In : Inport
  Discrete State-Space : DiscreteStateSpace  A=Ad  B=Bd  C=Cd  D=Dd  X0=x0d  SampleTime=Ts
  Out : Outport
  wires:
  In/1 -> Discrete State-Space/1
  Discrete State-Space/1 -> Out/1

== system Grid_1/GenSet_4MVA_09212015/900kW Generator with Primary Controllers/Diesel Engine Speed & Voltage Control fast/Excitation/Main Regulator ka // (ta.s +1) ==
  note: link disabled
  In : Inport
  1st order Lowpass : Subsystem  AncestorBlock=|  mask(Discrete 1st-Order Filter){FilterType=Lowpass, Tc=reg(2), Ts=Ts, Initialize=on, Vac_Init=[0.0 0 60], Vdc_Init=exc(1)*v0(2), PlotResponse=off, param1=[1 500 0.1]}
      | powerlib_extras/Discrete 
      | Control Blocks/Discrete
      | 1st-Order
      | Discrete Filter
      mask prompts: FilterType "Filter Type:"; Tc "Time constant (s):"; Ts "Sample time:"; Initialize "Initialize filter states"; Vac_Init "AC initial input: [ Mag  Phase(degrees)  Freq(Hz) ]"; Vdc_Init "DC Initial input:"; PlotResponse "Plot filter response"; param1 "Frequency range(Hz) : [Start  End  Inc.]"
      mask init: same as Grid_1/GenSet_1MVA_09082015/900kW Generator with Primary Controllers/Diesel Engine Speed & Voltage Control fast/Excitation/Low Pass Filter 1 / (tr.s +1) (with IC)
      mask TypeOptions FilterType: Lowpass | Highpass
      mask Callback Initialize: p4=get_param(gcb,'Initialize');if strcmp(p4,'on');visible={'on','on','on','on','on','on','on',get_param(gcb,'PlotResponse')};else;visible={'on','on','on','on','off','off','on',get_param(gcb,'PlotResponse')};end;set_param(gcb,'MaskVisibilities',visible)
      mask Callback PlotResponse: p7=get_param(gcb,'PlotResponse');if strcmp(p7,'on');visible={'on','on','on','on',get_param(gcb,'Initialize'),get_param(gcb,'Initialize'),'on','on'};else;visible={'on','on','on','on',get_param(gcb,'Initialize'),get_param(gcb,'Initialize'),'on','off'};end;set_param(gcb,'MaskVisibilities',visible)
      mask Display: plot(X,Y);
  Gain : Gain  Gain=reg(1)  SaturateOnIntegerOverflow=on  OutDataTypeStr=Inherit: Same as input  ParamDataTypeStr=Inherit: Same as input
  Out : Outport
  wires:
  1st order Lowpass/1(Out) -> Out/1
  In/1 -> Gain/1
  Gain/1 -> 1st order Lowpass/1(In)

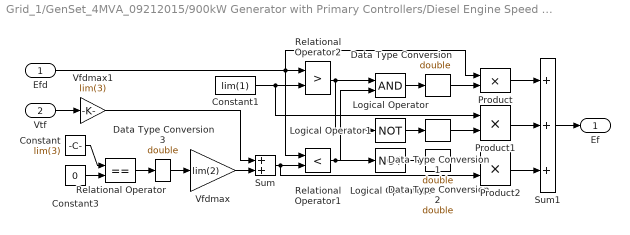
== system Grid_1/GenSet_4MVA_09212015/900kW Generator with Primary Controllers/Diesel Engine Speed & Voltage Control fast/Excitation/proportional saturation ==
  Efd : Inport
  Vtf : Inport  Port=2
  Constant : Constant  Value=lim(3)
  Constant1 : Constant  Value=lim(1)
  Constant3 : Constant  Value=0
  Data Type Conversion{,1..3} (4 alike) : DataTypeConversion  OutDataTypeStr=double  SaturateOnIntegerOverflow=on  RndMeth=Zero
  Logical Operator : Logic
  Logical Operator1 : Logic  Operator=NOT  Inputs=1
  Logical Operator2 : Logic  Operator=NOT  Inputs=1
  Product : Product  SaturateOnIntegerOverflow=on  InputSameDT=on  OutDataTypeStr=Inherit: Same as first input
  Product1 : Product  SaturateOnIntegerOverflow=on  InputSameDT=on  OutDataTypeStr=Inherit: Same as first input
  Product2 : Product  SaturateOnIntegerOverflow=on  InputSameDT=on  OutDataTypeStr=Inherit: Same as first input
  Relational Operator : RelationalOperator  Operator===  RndMeth=Nearest  InputSameDT=on
  Relational Operator1 : RelationalOperator  Operator=<  RndMeth=Nearest  InputSameDT=on
  Relational Operator2 : RelationalOperator  Operator=>  RndMeth=Nearest  InputSameDT=on
  Sum : Sum  SaturateOnIntegerOverflow=on  InputSameDT=on  OutDataTypeStr=Inherit: Same as first input
  Sum1 : Sum  Inputs=+++  SaturateOnIntegerOverflow=on  InputSameDT=on  OutDataTypeStr=Inherit: Same as first input
  Vfdmax : Gain  Gain=lim(2)  SaturateOnIntegerOverflow=on  OutDataTypeStr=Inherit: Same as input  ParamDataTypeStr=Inherit: Same as input
  Vfdmax1 : Gain  Gain=lim(3)  SaturateOnIntegerOverflow=on  OutDataTypeStr=Inherit: Same as input  ParamDataTypeStr=Inherit: Same as input
  Ef : Outport
  wires:
  Data Type Conversion3/1 -> Vfdmax/1
  Relational Operator/1 -> Data Type Conversion3/1
  Data Type Conversion2/1 -> Product2/1
  Logical Operator2/1 -> Data Type Conversion2/1
  Data Type Conversion1/1 -> Product1/2
  Logical Operator1/1 -> Data Type Conversion1/1
  Data Type Conversion/1 -> Product/2
  Logical Operator/1 -> Data Type Conversion/1
  Product1/1 -> Sum1/2
  Product2/1 -> Sum1/3
  Product/1 -> Sum1/1
  Sum1/1 -> Ef/1
  Efd/1 -> Product/1, Relational Operator1/1, Relational Operator2/1
  Constant1/1 -> Product1/1, Relational Operator2/2
  Relational Operator1/1 -> Logical Operator/2, Logical Operator2/1
  Relational Operator2/1 -> Logical Operator/1, Logical Operator1/1
  Sum/1 -> Relational Operator1/2, Product2/2
  Vfdmax1/1 -> Sum/1
  Vfdmax/1 -> Sum/2
  Constant3/1 -> Relational Operator/2
  Constant/1 -> Relational Operator/1
  Vtf/1 -> Vfdmax1/1

== system Grid_1/GenSet_1MVA_09082015/900kW Generator with Primary Controllers/Diesel Engine Speed & Voltage Control fast/Excitation/Damping kf.s // (tf.s +1)/1st-Order Discrete Filter ==
  In : Inport
  Discrete State-Space : DiscreteStateSpace  A=Ad  B=Bd  C=Cd  D=Dd  X0=x0d  SampleTime=Ts
  Out : Outport
  wires:
  Discrete State-Space/1 -> Out/1
  In/1 -> Discrete State-Space/1
